simulink model "queue_model"  (R2020b)
settings: Solver=FixedStepDiscrete  StartTime=0.0  StopTime=10.0  FixedStep=1  RelTol=1e-3
settings Model: Creator=rsub  LastModifiedBy=rsub

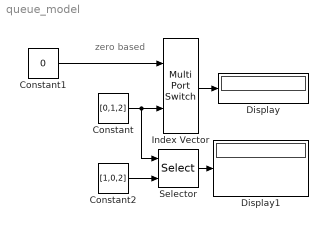
== system queue_model ==
  note: zero based
  Constant : Constant  Value=[0,1,2]
  Constant1 : Constant  Value=0
  Constant2 : Constant  Value=[1,0,2]
  Display : Display
  Display1 : Display
  Index Vector : MultiPortSwitch  DataPortOrder=Zero-based contiguous  Inputs=1  zeroidx=on
  Selector : Selector  IndexMode=Zero-based  InputPortWidth=3  IndexOptions=Index vector (port)  Indices=[1 3]  OutputSizes=1
  wires:
  Constant/1 -> Selector/1, Index Vector/2
  Index Vector/1 -> Display/1
  Constant1/1 -> Index Vector/1
  Constant2/1 -> Selector/2
  Selector/1 -> Display1/1
